simulink model "ex6_s"  (R2018b)
settings: Solver=VariableStepAuto  StartTime=0.0  StopTime=1000.0  RelTol=1e-3
values from neighbouring files (symbols this model uses):
  A = [-11 -2.5 0;4 0 0;0 0.25 0]    [ex1.m]    (also in ex2.m; ex3.m = sys_s.a; ex4.m = sys_s.A; ex5.m = sys_c.A)
  B = [4 0 0]'    [ex1.m]    (also in ex2.m; ex3.m = sys_s.b; ex4.m = sys_s.B; ex5.m = sys_c.B)
  k_d = 2    [ex2.m]    (also in ex3.m; ex4.m; ex5.m; ex6.m)
  k_i = Kt(4)    [ex4.m]    (also in ex5.m = T*Kt(4); ex6.m = T*Kt(4); motore_posizione.m)
  k_x = Kt(1:3)    [ex4.m]    (also in ex5.m; ex6.m; motore_posizione.m)
  T = 0.5/20    (= 0.025)    [ex3.m]    (also in ex5.m = 0.1; ex6.m = 0.2; ex8.m = 0.15; motore_posizione.m = 0.3)
settings Model: Creator=michelemaresca  LastModifiedBy=michelemaresca

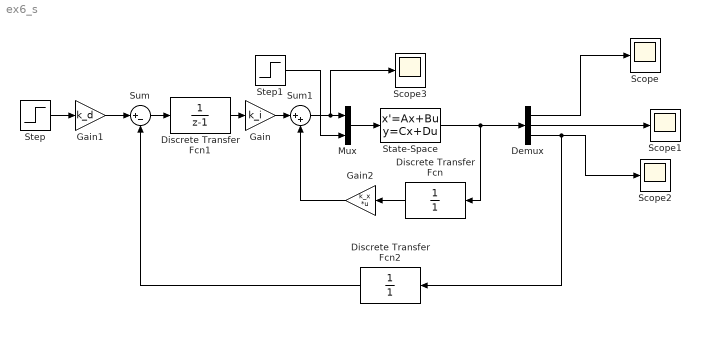
== system ex6_s ==
  Demux : Demux  Outputs=3
  Discrete Transfer Fcn : DiscreteTransferFcn  Denominator=[1]  SampleTime=T
  Discrete Transfer Fcn1 : DiscreteTransferFcn  Denominator=[1 -1]  SampleTime=T
  Discrete Transfer Fcn2 : DiscreteTransferFcn  Denominator=[1]  SampleTime=T
  Gain : Gain  Gain=k_i
  Gain1 : Gain  Gain=k_d
  Gain2 : Gain  Gain=k_x  Multiplication=Matrix(K*u)
  Mux : Mux  Inputs=2
  Scope{,1..3} (4 alike) : Scope
  State-Space : StateSpace  A=A  B=[B,[0;-1;0]]  C=eye(3)  D=zeros(3,2)  InitialCondition=0
  Step : Step  Time=0  SampleTime=T
  Step1 : Step  Time=500  After=5  SampleTime=T
  Sum : Sum  Inputs=|+-
  Sum1 : Sum  Inputs=|++
  wires:
  Demux/3 -> Discrete Transfer Fcn2/1, Scope2/1
  Discrete Transfer Fcn2/1 -> Sum/2
  Sum/1 -> Discrete Transfer Fcn1/1
  Sum1/1 -> Scope3/1, Mux/1
  Gain2/1 -> Sum1/2
  Demux/2 -> Scope1/1
  Demux/1 -> Scope/1
  Mux/1 -> State-Space/1
  Step1/1 -> Mux/2
  Gain/1 -> Sum1/1
  Step/1 -> Gain1/1
  State-Space/1 -> Demux/1, Discrete Transfer Fcn/1
  Discrete Transfer Fcn/1 -> Gain2/1
  Gain1/1 -> Sum/1
  Discrete Transfer Fcn1/1 -> Gain/1
